simulink model "Demo_V2XStats_Intersection_1_cs"  (R2014b)
settings: Solver=FixedStepDiscrete  SolverMode=SingleTasking  StartTime=0.0  StopTime=10  FixedStep=1/20  RelTol=1e-3
PreLoadFcn:
  | mbxruntime.callbacks.PreLoadFcn(bdroot);
  | check_NUTS_defined
  | model_closed = 0;
  | assignin('base',['model_closed_' bdroot],false);
PostLoadFcn:
  | mbxruntime.callbacks.PostLoadFcn(bdroot);
InitFcn:
  | mbxruntime.callbacks.InitFcn(bdroot);
StartFcn:
  | mbxruntime.callbacks.StartFcn(bdroot);
StopFcn:
  | mbxruntime.callbacks.StopFcn(bdroot);;
  | 
  | PostProcessing
  | 
model workspace: external: MAT-File .\Demo_V2XStats_Intersection_1_cs_hws.mat (data not in the file)
undefined symbols (not defined in the file or in its folder): InitializeBus, mbxruntime, tabledata
undefined symbols (not defined in the file): Demo_V2XStats_Intersection_1_cs_022fa72960d02a99, Demo_V2XStats_Intersection_1_cs_0667b7440011464a, Demo_V2XStats_Intersection_1_cs_0a717f3b1f82dce8, Demo_V2XStats_Intersection_1_cs_1912d0ac773e0614, Demo_V2XStats_Intersection_1_cs_1b4820430dd12493, Demo_V2XStats_Intersection_1_cs_3bba87328ee67e0a, Demo_V2XStats_Intersection_1_cs_467d7b57b3557fc2, Demo_V2XStats_Intersection_1_cs_534bad308c560994, Demo_V2XStats_Intersection_1_cs_58d6839509a0e403, Demo_V2XStats_Intersection_1_cs_7e2090151d7b4087, Demo_V2XStats_Intersection_1_cs_9888c4f7e8bf41a4, Demo_V2XStats_Intersection_1_cs_a103b1f27004d7b9, Demo_V2XStats_Intersection_1_cs_dde6e9b2bb85eae6, Demo_V2XStats_Intersection_1_cs_fcdd4688b7d5d124
libraries: simulink x5, PreScanSimulinkLibrary x4, PreScanUsefulBlocks x1, simulink_extras x1
(part 2 of 3)

== system Demo_V2XStats_Intersection_1_cs/Synchronizer ==
  Bus Selector1 : BusSelector  OutputSignals=FederateStopped
  Stop Simulation : Stop
  sfun_Synchronizer : S-Function  FunctionName=sfun_Synchronizer  Parameters=SampleTime  EnableBusSupport=off  mask(Legacy Function){SFunctionSpec=void prescan_synchronizer_outputFcn(void ** work1, PRESCAN_SYNCHRONIZEDATA y1[1]), SampleTime=TimeStep, ShowSpec=on}
      mask prompts: SampleTime "Sample time (-1 for inherited):"; ShowSpec "Display function specification"
      mask help:
      | This block allows you to call the legacy functions specified by the following Legacy Code Tool definition:
      | def.SFunctionName = 'sfun_Synchronizer';
      | def.OutputFcnSpec = 'void prescan_synchronizer_outputFcn(void ** work1, PRESCAN_SYNCHRONIZEDATA y1[1])';
      | def.StartFcnSpec = 'void prescan_synchronizer_startFcn(void ** work1)';
      | def.TerminateFcnSpec = 'void prescan_synchronizer_terminateFcn(void ** work1)';
      | def.HeaderFiles = {'prescan_synchronizer_data.h'};
      | def.HostLibFiles = {'sensorinterfaced.lib'};
      | def.IncPaths = {'src', 'C:\prescandev\vislibrary\vis\..\pimp\include\sensors\InterfaceRTW'};
      | def.SrcPaths = {'src'};
      | def.LibPaths = {'C:\\prescandev\\vislibrary_build\lib'};
      | def.SampleTime = 'parameterized';
      | def.Options.language = 'C';
      mask Help: <p>This block was generated automatically by the Legacy Code Tool. For detailed help on this tool, call<a href="matlab:legacy_code('help')"> legacy_code('help')</a>.</p>
      mask Callback ShowSpec:
      | if strcmp(get_param(gcbh, 'ShowSpec'), 'on')
      |   set_param(gcbh, 'MaskDisplay', sprintf('fprintf(''%s'');', get_param(gcbh, 'SFunctionSpec')));
      | else
      |   set_param(gcbh, 'MaskDisplay', sprintf('fprintf(''%s'');', get_param(gcbh, 'FunctionName')));
      | end
      mask Display: fprintf('void prescan_synchronizer_outputFcn(void ** work1, PRESCAN_SYNCHRONIZEDATA y1[1])');
  wires:
  Bus Selector1/1 -> Stop Simulation/1  "<FederateStopped>"
  sfun_Synchronizer/1 -> Bus Selector1/1

== system Demo_V2XStats_Intersection_1_cs/V2X_Rx2816_CAM_Receiver ==
  Sensor : S-Function  LoadFcn=InitializeBus('CAM')  FunctionName=sfun_V2X_CAM_Receiver  Parameters=sensorID, parentID, maxMessages, timestep  EnableBusSupport=off  mask(V2X CAM Receiver Block){sensorID=2816, parentID=7, maxMessages=1, timestep=1/20}
      mask prompts: sensorID "Receiver ID"; parentID "Parent ID"; maxMessages "Maximum number of messages"; timestep "MATLAB timestep:"
      mask help: V2X Block receiving a CAM message
      mask Display: image(imread('V2XR_grayscale.png'))
  V2X_Rx2816_CAM_Receiver : Outport  Tag=outport/plugin/sfun_V2X_CAM_Receiver
  wires:
  Sensor/1 -> V2X_Rx2816_CAM_Receiver/1

== system Demo_V2XStats_Intersection_1_cs/V2X_Tx2817_CAM_Transmitter ==
  V2X_Tx2817_CAM_Transmitter : Inport  Tag=inport/plugin/sfun_V2X_CAM_Transmitter  BusOutputAsStruct=on
  Actuator : S-Function  FunctionName=sfun_V2X_CAM_Transmitter  Parameters=sensorID, parentID, timestep  EnableBusSupport=off  mask(V2X CAM Transmitter Block){sensorID=2817, parentID=10, timestep=1/20}
      mask prompts: sensorID "Transmitter ID"; parentID "Parent ID"; timestep "MATLAB timestep:"
      mask help: V2X Block transmitting a CAM message
      mask Display: image(imread('V2XT_grayscale.png'))
  wires:
  V2X_Tx2817_CAM_Transmitter/1 -> Actuator/1

== system Demo_V2XStats_Intersection_1_cs/VISUColorRegion_Lower_Body_Male_Regular_wSuitcase_1 ==
  VISUColorRegion_Lower_Body_Male_Regular_wSuitcase_1 : Inport  Tag=inport/ColorRegion  OutDataTypeStr=Bus: PRESCAN_COLOR_DATA  PortDimensions=1  SampleTime=1/20  BusOutputAsStruct=on
  Actuator : S-Function  FunctionName=sfun_ColorActuator  Parameters=mbxruntime.parameters.convert(UniqueID), mbxruntime.parameters.convert(WorldModelSubPath),tabledata, TimeStep  EnableBusSupport=off  mask(PreScan Sink Block: VisuTextureColor){UniqueID=2658, WorldModelSubPath=/recolorRegion:name=Lower Body/targetColor, TimeStep=1/20}
      mask prompts: UniqueID "Parent Unique Identifier (auto-generated)"; WorldModelSubPath "WM SubPath(auto-generated)"; TimeStep "Simulink time step"
      mask help:
      | The VisuTextureColor block provides a way to adapt the color of a vehicle.
      |
      | For more information, please click Help.
      mask init:
      | [tabledata] = mbxruntime.parameters.table(UniqueID,WorldModelSubPath);
      mask Help: eval('openHelp(230)')
      mask Display: image(imread('TextureColor.png'))
  wires:
  VISUColorRegion_Lower_Body_Male_Regular_wSuitcase_1/1 -> Actuator/1

== system Demo_V2XStats_Intersection_1_cs/VISUColorRegion_Shoes_Male_Regular_wSuitcase_1 ==
  VISUColorRegion_Shoes_Male_Regular_wSuitcase_1 : Inport  Tag=inport/ColorRegion  OutDataTypeStr=Bus: PRESCAN_COLOR_DATA  PortDimensions=1  SampleTime=1/20  BusOutputAsStruct=on
  Actuator : S-Function  FunctionName=sfun_ColorActuator  Parameters=mbxruntime.parameters.convert(UniqueID), mbxruntime.parameters.convert(WorldModelSubPath),tabledata, TimeStep  EnableBusSupport=off  mask(PreScan Sink Block: VisuTextureColor){UniqueID=2658, WorldModelSubPath=/recolorRegion:name=Shoes/targetColor, TimeStep=1/20}
      mask prompts: UniqueID "Parent Unique Identifier (auto-generated)"; WorldModelSubPath "WM SubPath(auto-generated)"; TimeStep "Simulink time step"
      mask help:
      | The VisuTextureColor block provides a way to adapt the color of a vehicle.
      |
      | For more information, please click Help.
      mask init:
      | [tabledata] = mbxruntime.parameters.table(UniqueID,WorldModelSubPath);
      mask Help: eval('openHelp(230)')
      mask Display: image(imread('TextureColor.png'))
  wires:
  VISUColorRegion_Shoes_Male_Regular_wSuitcase_1/1 -> Actuator/1

== system Demo_V2XStats_Intersection_1_cs/VISUColorRegion_Upper_Body_Male_Regular_wSuitcase_1 ==
  VISUColorRegion_Upper_Body_Male_Regular_wSuitcase_1 : Inport  Tag=inport/ColorRegion  OutDataTypeStr=Bus: PRESCAN_COLOR_DATA  PortDimensions=1  SampleTime=1/20  BusOutputAsStruct=on
  Actuator : S-Function  FunctionName=sfun_ColorActuator  Parameters=mbxruntime.parameters.convert(UniqueID), mbxruntime.parameters.convert(WorldModelSubPath),tabledata, TimeStep  EnableBusSupport=off  mask(PreScan Sink Block: VisuTextureColor){UniqueID=2658, WorldModelSubPath=/recolorRegion:name=Upper Body/targetColor, TimeStep=1/20}
      mask prompts: UniqueID "Parent Unique Identifier (auto-generated)"; WorldModelSubPath "WM SubPath(auto-generated)"; TimeStep "Simulink time step"
      mask help:
      | The VisuTextureColor block provides a way to adapt the color of a vehicle.
      |
      | For more information, please click Help.
      mask init:
      | [tabledata] = mbxruntime.parameters.table(UniqueID,WorldModelSubPath);
      mask Help: eval('openHelp(230)')
      mask Display: image(imread('TextureColor.png'))
  wires:
  VISUColorRegion_Upper_Body_Male_Regular_wSuitcase_1/1 -> Actuator/1

== system Demo_V2XStats_Intersection_1_cs/Male_Regular_wSuitcase_1/Animation ==
  In1 : Inport
  Bus Creator : BusCreator  Inputs=2  OutDataTypeStr=Bus: PRESCAN_ANIMACTUATORDATA  NonVirtualBus=on
  Bus Selector : BusSelector  OutputSignals=VelocityX,VelocityY,VelocityZ
  Mux : Mux  Inputs=3
  animation mode : Subsystem
  elapsed track : Subsystem
  Out1 : Outport
  wires:
  animation mode/1(mode) -> Bus Creator/1  "Index"
  Bus Creator/1 -> Out1/1
  In1/1 -> Bus Selector/1
  elapsed track/1(s) -> Bus Creator/2  "Time"
  Bus Selector/3 -> Mux/3  "<VelocityZ>"
  Bus Selector/2 -> Mux/2  "<VelocityY>"
  Bus Selector/1 -> Mux/1  "<VelocityX>"
  Mux/1 -> animation mode/1(vel), elapsed track/1(vel)

== system Demo_V2XStats_Intersection_1_cs/Male_Regular_wSuitcase_1/Dynamics_Empty ==
  note: For state mode 'Dynamic' positions
      | are not taken into account, as they
      | are computed by integrating velocity.
      | Click annotation for Help.
  note: For state mode 'Dynamic' positions
      | are not taken into account, as they
      | are computed by integrating velocity.
      | Click annotation for Help.
  Ground_{1..9} (9 alike) : Ground
  MuxState : Subsystem  Tag=mux/State  mask(Empty Dynamics State Block){positioningmode=on, TimeStep=1/20}
      mask prompts: positioningmode "Positioning Mode"; TimeStep "Auto Assigned: Time Step [s]"
      mask help:
      | Build the state of an actor based on user input.
      | The user can either use positioning mode or dynamics mode.
      | - When using positioning mode the position and orientation of the actor are set directly based on the input. Expected input is relative to the initial position and orientation of the actor. It's also possible to specify the velocity of the actor, though this input isn't used, only passed on.
      | - When using dynamics mode the position input is ignored. Expected input is velocity and orientation. The velocity is relative the current orientation of the actor, while orientation is relative to its initial orientation. The position of the actor is calculated based on the velocity and orientation given.
      settings: DeleteFcn=PreScanBlockDeleteFcn;
  STATE_Male_Regular_wSuitcase_1 : Subsystem  Tag=mux/StatePort  Priority=0  LoadFcn=load PrescanStateActuatorData  mask(PreScan Sink Block: State){x0=Demo_V2XStats_Intersection_1_cs_9888c4f7e8bf41a4, y0=Demo_V2XStats_Intersection_1_cs_0667b7440011464a, z0=Demo_V2XStats_Intersection_1_cs_1b4820430dd12493, Roll0=Demo_V2XStats_Intersection_1_cs_dde6e9b2bb85eae6, Pitch0=Demo_V2XStats_Intersection_1_cs_1912d0ac773e0614, Yaw0=Demo_V2XStats_Intersection_1_cs_58d6839509a0e403, TimeStep=1/20}
      mask prompts: x0 "Ini x-position VEHICLE wrt GLOBAL axis system [m]"; y0 "Ini y-position VEHICLE wrt GLOBAL axis system [m]"; z0 "Ini z-position VEHICLE wrt GLOBAL axis system [m]"; Roll0 "Ini roll-angle BODY wrt VEHICLE axis system [deg]"; Pitch0 "Ini pitch-angle BODY wrt VEHICLE axis system [deg]"; Yaw0 "Ini yaw-angle VEHICLE wrt GLOBAL axis system [deg]"; TimeStep "Auto-Assigned: Upload Period [s]"
      mask help:
      | The Actor State contains a vector signal of size (9x1), containing the following signals:
      |
      | -  Position                  (x,y,z)                                     [m]
      | -  Velocity                  (vx,vy,vz)                               [m/s]
      | -  Angles                    (Roll, Pitch, Yaw)                   [rad]
      |
      | The Actor state is defined in the global axis system.
      | The state is superponed on the Initial position defined in the GUI.
      |
      | For more information, please click Help.
      settings: DeleteFcn=PreScanBlockDeleteFcn;
      mask Help: eval('openHelp(222)')
      mask Display: image(imread('State.png'))
  State : Outport  Tag=outport/StateOutport  SampleTime=1/20
  wires:
  STATE_Male_Regular_wSuitcase_1/1(StateBus) -> State/1
  MuxState/1(state) -> STATE_Male_Regular_wSuitcase_1/1(State)
  Ground_1/1 -> MuxState/1(x [m])
  Ground_2/1 -> MuxState/2(y [m])
  Ground_3/1 -> MuxState/3(z [m])
  Ground_4/1 -> MuxState/4(dx [m/s])
  Ground_5/1 -> MuxState/5(dy [m/s])
  Ground_6/1 -> MuxState/6(dz [m/s])
  Ground_7/1 -> MuxState/7(R [rad])
  Ground_8/1 -> MuxState/8(P [rad])
  Ground_9/1 -> MuxState/9(Y [rad])

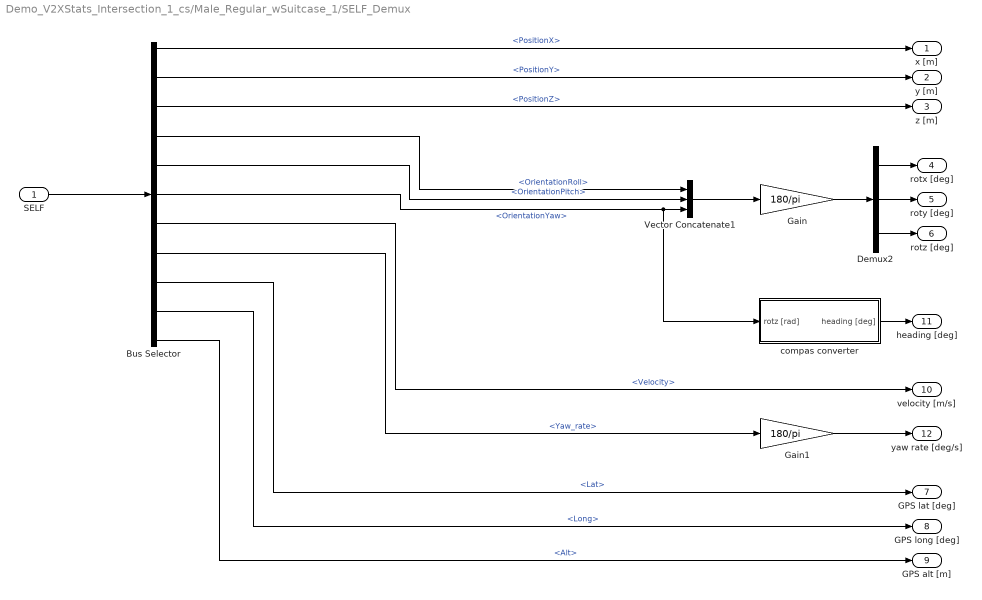
== system Demo_V2XStats_Intersection_1_cs/Male_Regular_wSuitcase_1/SELF_Demux ==
  SELF : Inport  OutDataTypeStr=Bus: PRESCAN_SELFSENSORDATA
  Bus Selector : BusSelector  OutputSignals=PositionX,PositionY,PositionZ,OrientationRoll,OrientationPitch,OrientationYaw,Velocity,Yaw_rate,Lat,Long,Alt
  Demux2 : Demux  Outputs=3
  Gain : Gain  Gain=180/pi
  Gain1 : Gain  Gain=180/pi
  Vector Concatenate1 : Concatenate  NumInputs=3
  compas converter : Subsystem
  x [m] : Outport
  y [m] : Outport  Port=2
  z [m] : Outport  Port=3
  rotx [deg] : Outport  Port=4
  roty [deg] : Outport  Port=5
  rotz [deg] : Outport  Port=6
  GPS lat [deg] : Outport  Port=7
  GPS long [deg] : Outport  Port=8
  GPS alt [m] : Outport  Port=9
  velocity [m/s] : Outport  Port=10
  heading [deg] : Outport  Port=11
  yaw rate [deg/s] : Outport  Port=12
  wires:
  Bus Selector/11 -> GPS alt [m]/1  "<Alt>"
  Bus Selector/10 -> GPS long [deg]/1  "<Long>"
  Bus Selector/9 -> GPS lat [deg]/1  "<Lat>"
  Bus Selector/8 -> Gain1/1  "<Yaw_rate>"
  Bus Selector/7 -> velocity [m/s]/1  "<Velocity>"
  Bus Selector/6 -> compas converter/1(rotz [rad]), Vector Concatenate1/3  "<OrientationYaw>"
  Bus Selector/5 -> Vector Concatenate1/2  "<OrientationPitch>"
  Bus Selector/4 -> Vector Concatenate1/1  "<OrientationRoll>"
  Vector Concatenate1/1 -> Gain/1
  Bus Selector/3 -> z [m]/1  "<PositionZ>"
  Bus Selector/2 -> y [m]/1  "<PositionY>"
  Bus Selector/1 -> x [m]/1  "<PositionX>"
  SELF/1 -> Bus Selector/1
  Gain/1 -> Demux2/1
  Demux2/1 -> rotx [deg]/1
  Demux2/2 -> roty [deg]/1
  Demux2/3 -> rotz [deg]/1
  compas converter/1(heading [deg]) -> heading [deg]/1
  Gain1/1 -> yaw rate [deg/s]/1

== system Demo_V2XStats_Intersection_1_cs/Male_Regular_wSuitcase_1/VISUColorRegion_Lower_Body_Mux ==
  RGB [-,-,-] : Inport
  Bus Creator : BusCreator  OutDataTypeStr=Bus: PRESCAN_COLOR_DATA  NonVirtualBus=on
  Constant : Constant  Value=255  OutDataTypeStr=uint8
  Data Type Conversion : DataTypeConversion  OutDataTypeStr=uint8
  Data Type Conversion1 : DataTypeConversion  OutDataTypeStr=uint8
  Data Type Conversion2 : DataTypeConversion  OutDataTypeStr=uint8
  Demux : Demux  Outputs=3
  ColorRegion : Outport  OutDataTypeStr=Bus: PRESCAN_COLOR_DATA  PortDimensions=1
  wires:
  Constant/1 -> Bus Creator/4  "A"
  Data Type Conversion2/1 -> Bus Creator/3  "B"
  Data Type Conversion1/1 -> Bus Creator/2  "G"
  Data Type Conversion/1 -> Bus Creator/1  "R"
  Demux/3 -> Data Type Conversion2/1  "B"
  Demux/2 -> Data Type Conversion1/1  "G"
  Demux/1 -> Data Type Conversion/1  "R"
  RGB [-,-,-]/1 -> Demux/1
  Bus Creator/1 -> ColorRegion/1

== system Demo_V2XStats_Intersection_1_cs/Male_Regular_wSuitcase_1/VISUColorRegion_Shoes_Mux ==
  RGB [-,-,-] : Inport
  Bus Creator : BusCreator  OutDataTypeStr=Bus: PRESCAN_COLOR_DATA  NonVirtualBus=on
  Constant : Constant  Value=255  OutDataTypeStr=uint8
  Data Type Conversion : DataTypeConversion  OutDataTypeStr=uint8
  Data Type Conversion1 : DataTypeConversion  OutDataTypeStr=uint8
  Data Type Conversion2 : DataTypeConversion  OutDataTypeStr=uint8
  Demux : Demux  Outputs=3
  ColorRegion : Outport  OutDataTypeStr=Bus: PRESCAN_COLOR_DATA  PortDimensions=1
  wires:
  Constant/1 -> Bus Creator/4  "A"
  Data Type Conversion2/1 -> Bus Creator/3  "B"
  Data Type Conversion1/1 -> Bus Creator/2  "G"
  Data Type Conversion/1 -> Bus Creator/1  "R"
  Demux/3 -> Data Type Conversion2/1  "B"
  Demux/2 -> Data Type Conversion1/1  "G"
  Demux/1 -> Data Type Conversion/1  "R"
  RGB [-,-,-]/1 -> Demux/1
  Bus Creator/1 -> ColorRegion/1

== system Demo_V2XStats_Intersection_1_cs/Male_Regular_wSuitcase_1/VISUColorRegion_Upper_Body_Mux ==
  RGB [-,-,-] : Inport
  Bus Creator : BusCreator  OutDataTypeStr=Bus: PRESCAN_COLOR_DATA  NonVirtualBus=on
  Constant : Constant  Value=255  OutDataTypeStr=uint8
  Data Type Conversion : DataTypeConversion  OutDataTypeStr=uint8
  Data Type Conversion1 : DataTypeConversion  OutDataTypeStr=uint8
  Data Type Conversion2 : DataTypeConversion  OutDataTypeStr=uint8
  Demux : Demux  Outputs=3
  ColorRegion : Outport  OutDataTypeStr=Bus: PRESCAN_COLOR_DATA  PortDimensions=1
  wires:
  Constant/1 -> Bus Creator/4  "A"
  Data Type Conversion2/1 -> Bus Creator/3  "B"
  Data Type Conversion1/1 -> Bus Creator/2  "G"
  Data Type Conversion/1 -> Bus Creator/1  "R"
  Demux/3 -> Data Type Conversion2/1  "B"
  Demux/2 -> Data Type Conversion1/1  "G"
  Demux/1 -> Data Type Conversion/1  "R"
  RGB [-,-,-]/1 -> Demux/1
  Bus Creator/1 -> ColorRegion/1

== system Demo_V2XStats_Intersection_1_cs/Mazda_RX8_1/Dynamics_Empty ==
  note: For state mode 'Dynamic' positions
      | are not taken into account, as they
      | are computed by integrating velocity.
      | Click annotation for Help.
  note: For state mode 'Dynamic' positions
      | are not taken into account, as they
      | are computed by integrating velocity.
      | Click annotation for Help.
  Ground_{1..9} (9 alike) : Ground
  MuxState : Subsystem  Tag=mux/State  mask(Empty Dynamics State Block){positioningmode=on, TimeStep=1/20}
      mask prompts: positioningmode "Positioning Mode"; TimeStep "Auto Assigned: Time Step [s]"
      mask help:
      | Build the state of an actor based on user input.
      | The user can either use positioning mode or dynamics mode.
      | - When using positioning mode the position and orientation of the actor are set directly based on the input. Expected input is relative to the initial position and orientation of the actor. It's also possible to specify the velocity of the actor, though this input isn't used, only passed on.
      | - When using dynamics mode the position input is ignored. Expected input is velocity and orientation. The velocity is relative the current orientation of the actor, while orientation is relative to its initial orientation. The position of the actor is calculated based on the velocity and orientation given.
      settings: DeleteFcn=PreScanBlockDeleteFcn;
  STATE_Mazda_RX8_1 : Subsystem  Tag=mux/StatePort  Priority=0  LoadFcn=load PrescanStateActuatorData  mask(PreScan Sink Block: State){x0=Demo_V2XStats_Intersection_1_cs_7e2090151d7b4087, y0=Demo_V2XStats_Intersection_1_cs_534bad308c560994, z0=Demo_V2XStats_Intersection_1_cs_467d7b57b3557fc2, Roll0=Demo_V2XStats_Intersection_1_cs_0a717f3b1f82dce8, Pitch0=Demo_V2XStats_Intersection_1_cs_3bba87328ee67e0a, Yaw0=Demo_V2XStats_Intersection_1_cs_022fa72960d02a99, TimeStep=1/20}
      mask prompts: x0 "Ini x-position VEHICLE wrt GLOBAL axis system [m]"; y0 "Ini y-position VEHICLE wrt GLOBAL axis system [m]"; z0 "Ini z-position VEHICLE wrt GLOBAL axis system [m]"; Roll0 "Ini roll-angle BODY wrt VEHICLE axis system [deg]"; Pitch0 "Ini pitch-angle BODY wrt VEHICLE axis system [deg]"; Yaw0 "Ini yaw-angle VEHICLE wrt GLOBAL axis system [deg]"; TimeStep "Auto-Assigned: Upload Period [s]"
      mask help:
      | The Actor State contains a vector signal of size (9x1), containing the following signals:
      |
      | -  Position                  (x,y,z)                                     [m]
      | -  Velocity                  (vx,vy,vz)                               [m/s]
      | -  Angles                    (Roll, Pitch, Yaw)                   [rad]
      |
      | The Actor state is defined in the global axis system.
      | The state is superponed on the Initial position defined in the GUI.
      |
      | For more information, please click Help.
      settings: DeleteFcn=PreScanBlockDeleteFcn;
      mask Help: eval('openHelp(222)')
      mask Display: image(imread('State.png'))
  State : Outport  Tag=outport/StateOutport  SampleTime=1/20
  wires:
  STATE_Mazda_RX8_1/1(StateBus) -> State/1
  MuxState/1(state) -> STATE_Mazda_RX8_1/1(State)
  Ground_1/1 -> MuxState/1(x [m])
  Ground_2/1 -> MuxState/2(y [m])
  Ground_3/1 -> MuxState/3(z [m])
  Ground_4/1 -> MuxState/4(dx [m/s])
  Ground_5/1 -> MuxState/5(dy [m/s])
  Ground_6/1 -> MuxState/6(dz [m/s])
  Ground_7/1 -> MuxState/7(R [rad])
  Ground_8/1 -> MuxState/8(P [rad])
  Ground_9/1 -> MuxState/9(Y [rad])

== system Demo_V2XStats_Intersection_1_cs/Mazda_RX8_1/Retreive car data using ID info ==
  note: id=4
  note: id=4
  note: Assumption:
      | All vehicles are visible all time.
      | So the data can be ordered by using the id order.
      | id=0 (meaning no detection) does not exist
  Lat_detected : Inport
  Lon_detected : Inport  Port=2
  Alt_detected : Inport  Port=3
  Intention_detected : Inport  Port=4
  Heading_detected : Inport  Port=5
  Complex to Magnitude-Angle1 : ComplexToMagnitudeAngle
  Demux1 : Demux  Outputs=2
  GPS2xyz : PreScanUsefulBlocks/GPS2xyz  CoordinateCount=1  GPS_base=[0 0 0]
  Mux : Mux
  Mux3 : Mux  Inputs=3
  Radians to Degrees : simulink_extras/Transformations/Radians to Degrees
  Real-Imag to Complex1 : RealImagToComplex
  Selector : Selector  Indices=[1 2]
  Cabstar : Outport
  wires:
  Heading_detected/1 -> Mux/4  "heading"
  Intention_detected/1 -> Mux/3  "intention"
  Alt_detected/1 -> Mux3/3
  Lon_detected/1 -> Mux3/2
  Lat_detected/1 -> Mux3/1
  Mux/1 -> Cabstar/1
  Mux3/1 -> GPS2xyz/1
  Demux1/2 -> Real-Imag to Complex1/2
  Demux1/1 -> Real-Imag to Complex1/1
  Real-Imag to Complex1/1 -> Complex to Magnitude-Angle1/1
  Complex to Magnitude-Angle1/2 -> Radians to Degrees/1
  Radians to Degrees/1 -> Mux/2  "angle"
  Complex to Magnitude-Angle1/1 -> Mux/1  "range"
  Selector/1 -> Demux1/1
  GPS2xyz/1 -> Selector/1

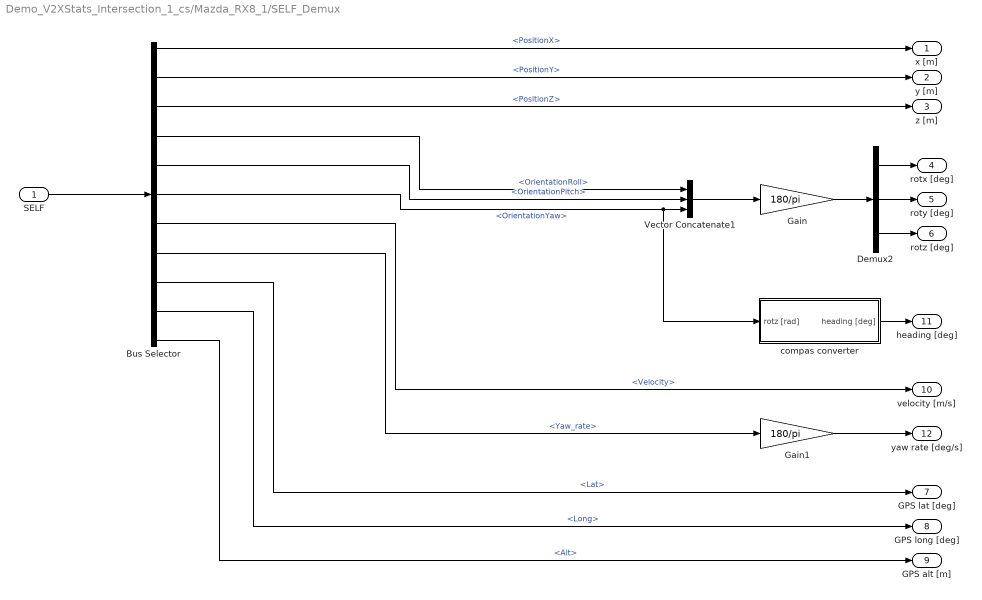
== system Demo_V2XStats_Intersection_1_cs/Mazda_RX8_1/SELF_Demux ==
  SELF : Inport  OutDataTypeStr=Bus: PRESCAN_SELFSENSORDATA
  Bus Selector : BusSelector  OutputSignals=PositionX,PositionY,PositionZ,OrientationRoll,OrientationPitch,OrientationYaw,Velocity,Yaw_rate,Lat,Long,Alt
  Demux2 : Demux  Outputs=3
  Gain : Gain  Gain=180/pi
  Gain1 : Gain  Gain=180/pi
  Vector Concatenate1 : Concatenate  NumInputs=3
  compas converter : Subsystem
  x [m] : Outport
  y [m] : Outport  Port=2
  z [m] : Outport  Port=3
  rotx [deg] : Outport  Port=4
  roty [deg] : Outport  Port=5
  rotz [deg] : Outport  Port=6
  GPS lat [deg] : Outport  Port=7
  GPS long [deg] : Outport  Port=8
  GPS alt [m] : Outport  Port=9
  velocity [m/s] : Outport  Port=10
  heading [deg] : Outport  Port=11
  yaw rate [deg/s] : Outport  Port=12
  wires:
  Bus Selector/11 -> GPS alt [m]/1  "<Alt>"
  Bus Selector/10 -> GPS long [deg]/1  "<Long>"
  Bus Selector/9 -> GPS lat [deg]/1  "<Lat>"
  Bus Selector/8 -> Gain1/1  "<Yaw_rate>"
  Bus Selector/7 -> velocity [m/s]/1  "<Velocity>"
  Bus Selector/6 -> compas converter/1(rotz [rad]), Vector Concatenate1/3  "<OrientationYaw>"
  Bus Selector/5 -> Vector Concatenate1/2  "<OrientationPitch>"
  Bus Selector/4 -> Vector Concatenate1/1  "<OrientationRoll>"
  Vector Concatenate1/1 -> Gain/1
  Bus Selector/3 -> z [m]/1  "<PositionZ>"
  Bus Selector/2 -> y [m]/1  "<PositionY>"
  Bus Selector/1 -> x [m]/1  "<PositionX>"
  SELF/1 -> Bus Selector/1
  Gain/1 -> Demux2/1
  Demux2/1 -> rotx [deg]/1
  Demux2/2 -> roty [deg]/1
  Demux2/3 -> rotz [deg]/1
  compas converter/1(heading [deg]) -> heading [deg]/1
  Gain1/1 -> yaw rate [deg/s]/1

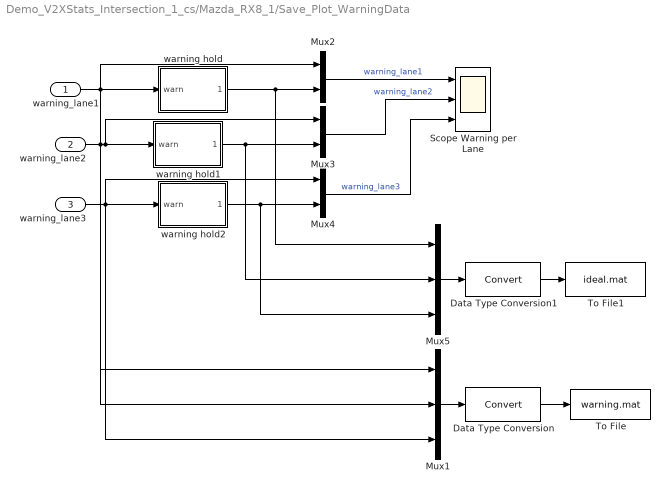
== system Demo_V2XStats_Intersection_1_cs/Mazda_RX8_1/Save_Plot_WarningData ==
  warning_lane1 : Inport
  warning_lane2 : Inport  Port=2
  warning_lane3 : Inport  Port=3
  Data Type Conversion : DataTypeConversion
  Data Type Conversion1 : DataTypeConversion
  Mux1 : Mux  Inputs=3
  Mux2 : Mux  Inputs=2
  Mux3 : Mux  Inputs=2
  Mux4 : Mux  Inputs=2
  Mux5 : Mux  Inputs=3
  Scope Warning per Lane : Scope  NumInputPorts=3
      settings: YMin=-5~-5~-5  YMax=5~5~5
  To File : ToFile  Filename=warning.mat  MatrixName=warning
  To File1 : ToFile  Filename=ideal.mat  MatrixName=ideal
  warning hold : Subsystem
  warning hold1 : Subsystem
  warning hold2 : Subsystem
  wires:
  Mux1/1 -> Data Type Conversion/1
  warning_lane3/1 -> Mux1/3, warning hold2/1(warn), Mux4/1
  warning_lane2/1 -> Mux1/2, warning hold1/1(warn), Mux3/1
  warning_lane1/1 -> Mux1/1, Mux2/1, warning hold/1(warn)
  Data Type Conversion1/1 -> To File1/1
  Mux5/1 -> Data Type Conversion1/1
  Data Type Conversion/1 -> To File/1
  Mux4/1 -> Scope Warning per Lane/3  "warning_lane3"
  Mux3/1 -> Scope Warning per Lane/2  "warning_lane2"
  Mux2/1 -> Scope Warning per Lane/1  "warning_lane1"
  warning hold2/1(warning) -> Mux5/3, Mux4/2
  warning hold1/1(warning) -> Mux5/2, Mux3/2
  warning hold/1(warning) -> Mux5/1, Mux2/2

== system Demo_V2XStats_Intersection_1_cs/Mazda_RX8_1/V2x_TC_GUI1 ==
  warning : Inport
  message : Inport  Port=2
  velocity : Inport  Port=3
  Constant : Constant  Value=800
  Constant2 : Constant  Value=0
  Constant3 : Constant  Value=0
  Data Type Conversion : DataTypeConversion
  Data Type Conversion1 : DataTypeConversion
  Detect Change : simulink/Logic and Bit Operations/Detect Change  vinit=0  InputProcessing=Inherited  OutDataTypeStr=uint8
  V2x_TC_GUI : M-S-Function  FunctionName=msfcn_V2x_TC_GUI
      mask Display:
      | port_label('input', 1, 'RPM');
      | port_label('input', 2, 'Velocity');
      | port_label('input', 3, 'Brake');
      | port_label('input', 4, 'Throttle');
      | port_label('input', 5, 'Message');
      | port_label('input', 6, 'Change');
      | port_label('input', 7, 'Warning');
  "[ms to kmh]" : Gain  Gain=3.6
  wires:
  "[ms to kmh]"/1 -> V2x_TC_GUI/2
  Constant3/1 -> V2x_TC_GUI/4
  Constant2/1 -> V2x_TC_GUI/3
  velocity/1 -> "[ms to kmh]"/1
  Constant/1 -> V2x_TC_GUI/1
  Data Type Conversion1/1 -> V2x_TC_GUI/7
  warning/1 -> Data Type Conversion1/1, Detect Change/1
  Data Type Conversion/1 -> V2x_TC_GUI/6
  Detect Change/1 -> Data Type Conversion/1
  message/1 -> V2x_TC_GUI/5

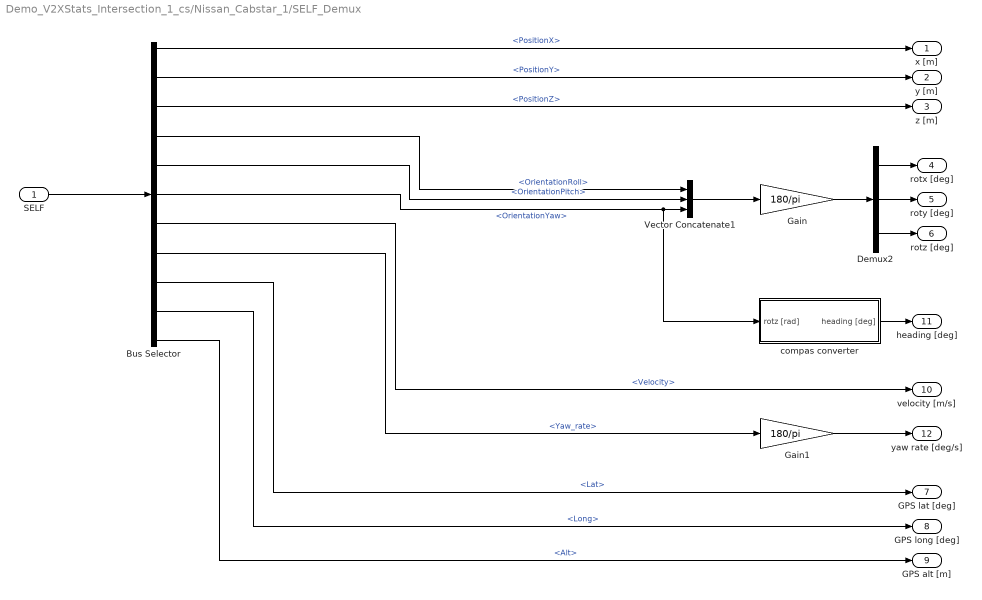
== system Demo_V2XStats_Intersection_1_cs/Nissan_Cabstar_1/SELF_Demux ==
  SELF : Inport  OutDataTypeStr=Bus: PRESCAN_SELFSENSORDATA
  Bus Selector : BusSelector  OutputSignals=PositionX,PositionY,PositionZ,OrientationRoll,OrientationPitch,OrientationYaw,Velocity,Yaw_rate,Lat,Long,Alt
  Demux2 : Demux  Outputs=3
  Gain : Gain  Gain=180/pi
  Gain1 : Gain  Gain=180/pi
  Vector Concatenate1 : Concatenate  NumInputs=3
  compas converter : Subsystem
  x [m] : Outport
  y [m] : Outport  Port=2
  z [m] : Outport  Port=3
  rotx [deg] : Outport  Port=4
  roty [deg] : Outport  Port=5
  rotz [deg] : Outport  Port=6
  GPS lat [deg] : Outport  Port=7
  GPS long [deg] : Outport  Port=8
  GPS alt [m] : Outport  Port=9
  velocity [m/s] : Outport  Port=10
  heading [deg] : Outport  Port=11
  yaw rate [deg/s] : Outport  Port=12
  wires:
  Bus Selector/11 -> GPS alt [m]/1  "<Alt>"
  Bus Selector/10 -> GPS long [deg]/1  "<Long>"
  Bus Selector/9 -> GPS lat [deg]/1  "<Lat>"
  Bus Selector/8 -> Gain1/1  "<Yaw_rate>"
  Bus Selector/7 -> velocity [m/s]/1  "<Velocity>"
  Bus Selector/6 -> compas converter/1(rotz [rad]), Vector Concatenate1/3  "<OrientationYaw>"
  Bus Selector/5 -> Vector Concatenate1/2  "<OrientationPitch>"
  Bus Selector/4 -> Vector Concatenate1/1  "<OrientationRoll>"
  Vector Concatenate1/1 -> Gain/1
  Bus Selector/3 -> z [m]/1  "<PositionZ>"
  Bus Selector/2 -> y [m]/1  "<PositionY>"
  Bus Selector/1 -> x [m]/1  "<PositionX>"
  SELF/1 -> Bus Selector/1
  Gain/1 -> Demux2/1
  Demux2/1 -> rotx [deg]/1
  Demux2/2 -> roty [deg]/1
  Demux2/3 -> rotz [deg]/1
  compas converter/1(heading [deg]) -> heading [deg]/1
  Gain1/1 -> yaw rate [deg/s]/1

== system Demo_V2XStats_Intersection_1_cs/Male_Regular_wSuitcase_1/Animation/animation mode ==
  vel : Inport
  Data Type Conversion : DataTypeConversion  OutDataTypeStr=int32
  Fcn : Fcn  Expr=u(1)^2+u(2)^2+u(3)^2
  Walking : simulink/Logic and Bit Operations/Compare To Zero  relop=~=  OutDataTypeStr=uint8  ZeroCross=off
  mode : Outport
  wires:
  Data Type Conversion/1 -> mode/1
  Walking/1 -> Data Type Conversion/1
  Fcn/1 -> Walking/1
  vel/1 -> Fcn/1

== system Demo_V2XStats_Intersection_1_cs/Male_Regular_wSuitcase_1/Animation/elapsed track ==
  vel : Inport
  Discrete-Time Integrator : DiscreteIntegrator  SampleTime=-1
  Fcn : Fcn  Expr=sqrt(u(1)^2 + u(2)^2 + u(3)^2)
  s : Outport
  wires:
  Discrete-Time Integrator/1 -> s/1
  vel/1 -> Fcn/1
  Fcn/1 -> Discrete-Time Integrator/1

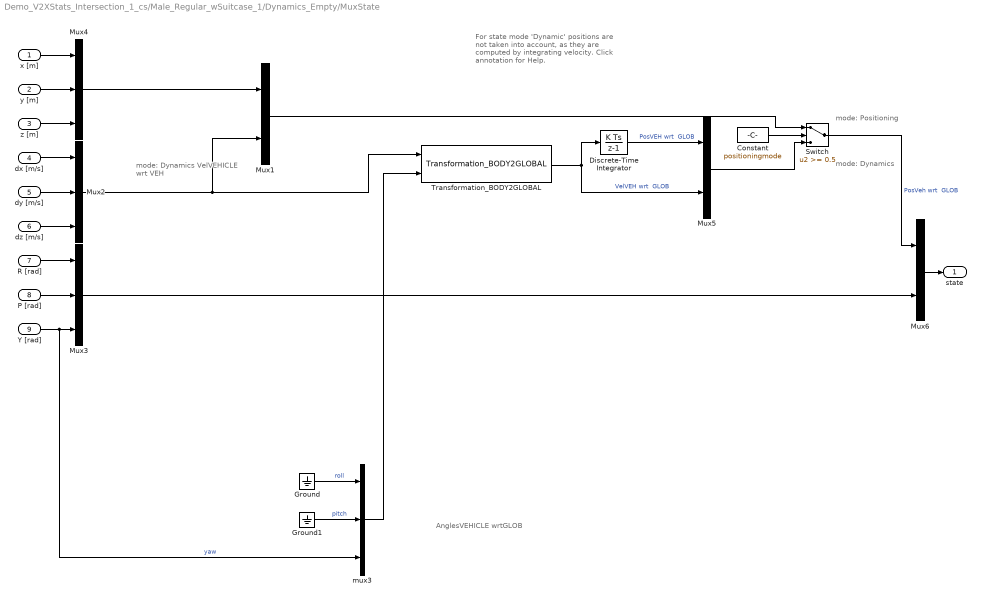
== system Demo_V2XStats_Intersection_1_cs/Male_Regular_wSuitcase_1/Dynamics_Empty/MuxState ==
  note: mode: Dynamics
  note: mode: Positioning
  note: mode: Dynamics
      | VelVEHICLE
      | wrt VEH
  note: AnglesVEHICLE
      | wrtGLOB
  note: For state mode 'Dynamic' positions
      | are not taken into account, as they
      | are computed by integrating velocity.
      | Click annotation for Help.
  x [m] : Inport  SampleTime=TimeStep
  y [m] : Inport  Port=2  SampleTime=TimeStep
  z [m] : Inport  Port=3  SampleTime=TimeStep
  dx [m/s] : Inport  Port=4  SampleTime=TimeStep
  dy [m/s] : Inport  Port=5  SampleTime=TimeStep
  dz [m/s] : Inport  Port=6  SampleTime=TimeStep
  R [rad] : Inport  Port=7  SampleTime=TimeStep
  P [rad] : Inport  Port=8  SampleTime=TimeStep
  Y [rad] : Inport  Port=9  SampleTime=TimeStep
  Constant : Constant  DisableCoverage=on  Value=positioningmode
  Discrete-Time Integrator : DiscreteIntegrator  SampleTime=TimeStep
  Ground : Ground
  Ground1 : Ground
  Mux1 : Mux  Inputs=[3 3]
  Mux2 : Mux  Inputs=3
  Mux3 : Mux  Inputs=3
  Mux4 : Mux  Inputs=3
  Mux5 : Mux  Inputs=[3 3]
  Mux6 : Mux  Inputs=[6 3]
  Switch : Switch  Threshold=0.5
  Transformation_BODY2GLOBAL : PreScanSimulinkLibrary/Simple_Vehicle_Dynamics/Chassis/MuxDynState/Transformation_BODY2GLOBAL
  mux3 : Mux  Inputs=3
  state : Outport
  wires:
  Constant/1 -> Switch/2
  Mux6/1 -> state/1
  Mux4/1 -> Mux1/1
  Mux5/1 -> Switch/3
  Mux1/1 -> Switch/1
  Switch/1 -> Mux6/1  "PosVeh wrt  GLOB"
  P [rad]/1 -> Mux3/2
  R [rad]/1 -> Mux3/1
  dz [m/s]/1 -> Mux2/3
  dy [m/s]/1 -> Mux2/2
  dx [m/s]/1 -> Mux2/1
  z [m]/1 -> Mux4/3
  y [m]/1 -> Mux4/2
  x [m]/1 -> Mux4/1
  Ground1/1 -> mux3/2  "pitch"
  Y [rad]/1 -> mux3/3, Mux3/3  "yaw"
  Mux3/1 -> Mux6/2
  Transformation_BODY2GLOBAL/1 -> Discrete-Time Integrator/1, Mux5/2  "VelVEH wrt  GLOB"
  mux3/1 -> Transformation_BODY2GLOBAL/2
  Ground/1 -> mux3/1  "roll"
  Mux2/1 -> Mux1/2, Transformation_BODY2GLOBAL/1
  Discrete-Time Integrator/1 -> Mux5/1  "PosVEH wrt  GLOB"

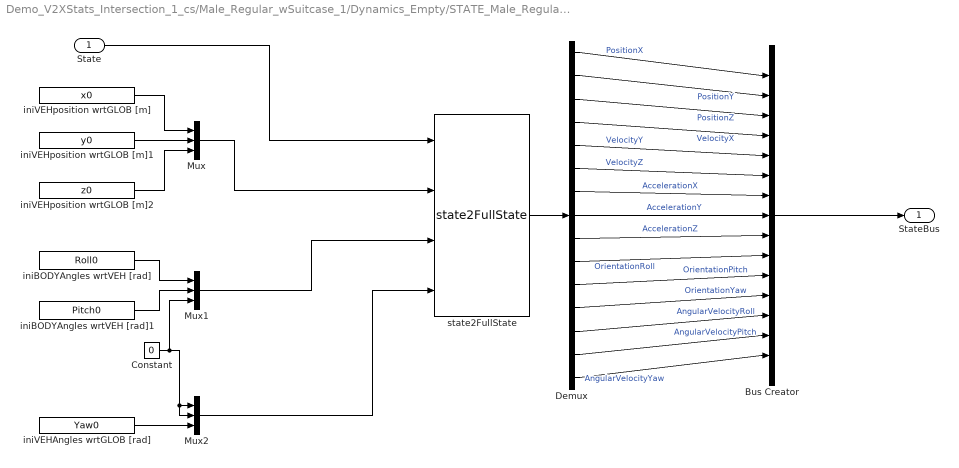
== system Demo_V2XStats_Intersection_1_cs/Male_Regular_wSuitcase_1/Dynamics_Empty/STATE_Male_Regular_wSuitcase_1 ==
  State : Inport  SampleTime=TimeStep
  Bus Creator : BusCreator  Inputs=15  OutDataTypeStr=Bus: PRESCAN_STATEACTUATORDATA  NonVirtualBus=on
  Constant : Constant  Value=0
  Demux : Demux  Outputs=15
  Mux : Mux  Inputs=3
  Mux1 : Mux  Inputs=3
  Mux2 : Mux  Inputs=3
  iniBODYAngles wrtVEH [rad] : Constant  Value=Roll0  SampleTime=TimeStep
  iniBODYAngles wrtVEH [rad]1 : Constant  Value=Pitch0  SampleTime=TimeStep
  iniVEHAngles wrtGLOB [rad] : Constant  Value=Yaw0  SampleTime=TimeStep
  iniVEHposition wrtGLOB [m] : Constant  Value=x0  SampleTime=TimeStep
  iniVEHposition wrtGLOB [m]1 : Constant  Value=y0  SampleTime=TimeStep
  iniVEHposition wrtGLOB [m]2 : Constant  Value=z0  SampleTime=TimeStep
  state2FullState : PreScanSimulinkLibrary/state2FullState  SystemSampleTime=-1
  StateBus : Outport  OutDataTypeStr=Bus: PRESCAN_STATEACTUATORDATA
  wires:
  Mux2/1 -> state2FullState/4
  iniVEHAngles wrtGLOB [rad]/1 -> Mux2/3
  Mux1/1 -> state2FullState/3
  Constant/1 -> Mux2/1, Mux2/2, Mux1/3
  iniBODYAngles wrtVEH [rad]1/1 -> Mux1/2
  iniBODYAngles wrtVEH [rad]/1 -> Mux1/1
  Mux/1 -> state2FullState/2
  iniVEHposition wrtGLOB [m]2/1 -> Mux/3
  iniVEHposition wrtGLOB [m]/1 -> Mux/1
  iniVEHposition wrtGLOB [m]1/1 -> Mux/2
  Demux/15 -> Bus Creator/15  "AngularVelocityYaw"
  Demux/14 -> Bus Creator/14  "AngularVelocityPitch"
  Demux/13 -> Bus Creator/13  "AngularVelocityRoll"
  Demux/12 -> Bus Creator/12  "OrientationYaw"
  Demux/11 -> Bus Creator/11  "OrientationPitch"
  Demux/10 -> Bus Creator/10  "OrientationRoll"
  Demux/9 -> Bus Creator/9  "AccelerationZ"
  Demux/8 -> Bus Creator/8  "AccelerationY"
  Demux/7 -> Bus Creator/7  "AccelerationX"
  Demux/6 -> Bus Creator/6  "VelocityZ"
  Demux/5 -> Bus Creator/5  "VelocityY"
  Demux/4 -> Bus Creator/4  "VelocityX"
  Demux/3 -> Bus Creator/3  "PositionZ"
  Demux/2 -> Bus Creator/2  "PositionY"
  Demux/1 -> Bus Creator/1  "PositionX"
  state2FullState/1 -> Demux/1
  State/1 -> state2FullState/1
  Bus Creator/1 -> StateBus/1

== system Demo_V2XStats_Intersection_1_cs/Male_Regular_wSuitcase_1/SELF_Demux/compas converter ==
  rotz [rad] : Inport
  cart2compas : Subsystem
  rad2deg : Gain  Gain=180/pi
  heading [deg] : Outport
  wires:
  rad2deg/1 -> cart2compas/1(Angle [deg])
  rotz [rad]/1 -> rad2deg/1
  cart2compas/1(heading [deg]) -> heading [deg]/1

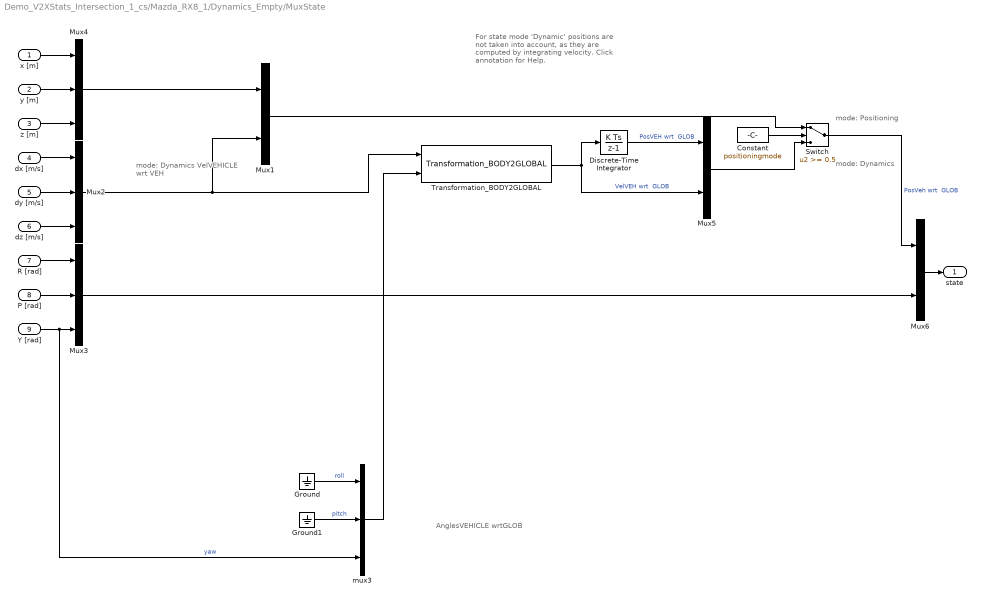
== system Demo_V2XStats_Intersection_1_cs/Mazda_RX8_1/Dynamics_Empty/MuxState ==
  note: mode: Dynamics
  note: mode: Positioning
  note: mode: Dynamics
      | VelVEHICLE
      | wrt VEH
  note: AnglesVEHICLE
      | wrtGLOB
  note: For state mode 'Dynamic' positions
      | are not taken into account, as they
      | are computed by integrating velocity.
      | Click annotation for Help.
  x [m] : Inport  SampleTime=TimeStep
  y [m] : Inport  Port=2  SampleTime=TimeStep
  z [m] : Inport  Port=3  SampleTime=TimeStep
  dx [m/s] : Inport  Port=4  SampleTime=TimeStep
  dy [m/s] : Inport  Port=5  SampleTime=TimeStep
  dz [m/s] : Inport  Port=6  SampleTime=TimeStep
  R [rad] : Inport  Port=7  SampleTime=TimeStep
  P [rad] : Inport  Port=8  SampleTime=TimeStep
  Y [rad] : Inport  Port=9  SampleTime=TimeStep
  Constant : Constant  DisableCoverage=on  Value=positioningmode
  Discrete-Time Integrator : DiscreteIntegrator  SampleTime=TimeStep
  Ground : Ground
  Ground1 : Ground
  Mux1 : Mux  Inputs=[3 3]
  Mux2 : Mux  Inputs=3
  Mux3 : Mux  Inputs=3
  Mux4 : Mux  Inputs=3
  Mux5 : Mux  Inputs=[3 3]
  Mux6 : Mux  Inputs=[6 3]
  Switch : Switch  Threshold=0.5
  Transformation_BODY2GLOBAL : PreScanSimulinkLibrary/Simple_Vehicle_Dynamics/Chassis/MuxDynState/Transformation_BODY2GLOBAL
  mux3 : Mux  Inputs=3
  state : Outport
  wires:
  Constant/1 -> Switch/2
  Mux6/1 -> state/1
  Mux4/1 -> Mux1/1
  Mux5/1 -> Switch/3
  Mux1/1 -> Switch/1
  Switch/1 -> Mux6/1  "PosVeh wrt  GLOB"
  P [rad]/1 -> Mux3/2
  R [rad]/1 -> Mux3/1
  dz [m/s]/1 -> Mux2/3
  dy [m/s]/1 -> Mux2/2
  dx [m/s]/1 -> Mux2/1
  z [m]/1 -> Mux4/3
  y [m]/1 -> Mux4/2
  x [m]/1 -> Mux4/1
  Ground1/1 -> mux3/2  "pitch"
  Y [rad]/1 -> mux3/3, Mux3/3  "yaw"
  Mux3/1 -> Mux6/2
  Transformation_BODY2GLOBAL/1 -> Discrete-Time Integrator/1, Mux5/2  "VelVEH wrt  GLOB"
  mux3/1 -> Transformation_BODY2GLOBAL/2
  Ground/1 -> mux3/1  "roll"
  Mux2/1 -> Mux1/2, Transformation_BODY2GLOBAL/1
  Discrete-Time Integrator/1 -> Mux5/1  "PosVEH wrt  GLOB"

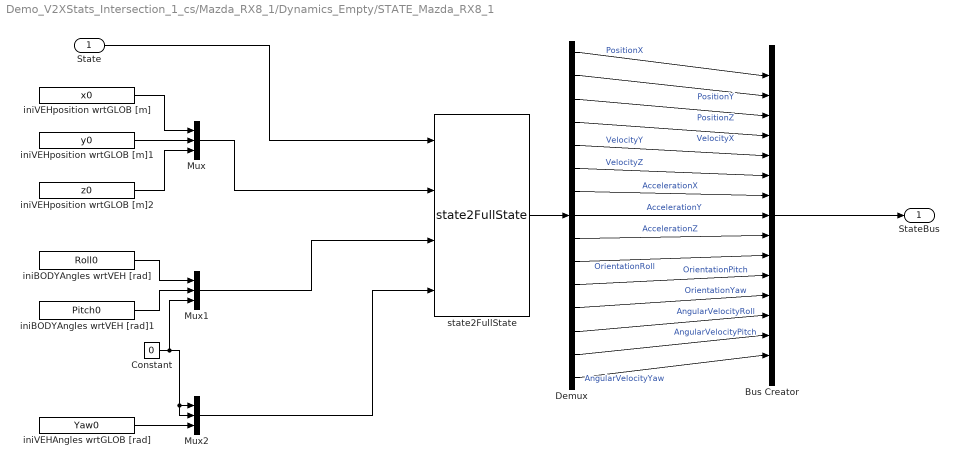
== system Demo_V2XStats_Intersection_1_cs/Mazda_RX8_1/Dynamics_Empty/STATE_Mazda_RX8_1 ==
  State : Inport  SampleTime=TimeStep
  Bus Creator : BusCreator  Inputs=15  OutDataTypeStr=Bus: PRESCAN_STATEACTUATORDATA  NonVirtualBus=on
  Constant : Constant  Value=0
  Demux : Demux  Outputs=15
  Mux : Mux  Inputs=3
  Mux1 : Mux  Inputs=3
  Mux2 : Mux  Inputs=3
  iniBODYAngles wrtVEH [rad] : Constant  Value=Roll0  SampleTime=TimeStep
  iniBODYAngles wrtVEH [rad]1 : Constant  Value=Pitch0  SampleTime=TimeStep
  iniVEHAngles wrtGLOB [rad] : Constant  Value=Yaw0  SampleTime=TimeStep
  iniVEHposition wrtGLOB [m] : Constant  Value=x0  SampleTime=TimeStep
  iniVEHposition wrtGLOB [m]1 : Constant  Value=y0  SampleTime=TimeStep
  iniVEHposition wrtGLOB [m]2 : Constant  Value=z0  SampleTime=TimeStep
  state2FullState : PreScanSimulinkLibrary/state2FullState  SystemSampleTime=-1
  StateBus : Outport  OutDataTypeStr=Bus: PRESCAN_STATEACTUATORDATA
  wires:
  Mux2/1 -> state2FullState/4
  iniVEHAngles wrtGLOB [rad]/1 -> Mux2/3
  Mux1/1 -> state2FullState/3
  Constant/1 -> Mux2/1, Mux2/2, Mux1/3
  iniBODYAngles wrtVEH [rad]1/1 -> Mux1/2
  iniBODYAngles wrtVEH [rad]/1 -> Mux1/1
  Mux/1 -> state2FullState/2
  iniVEHposition wrtGLOB [m]2/1 -> Mux/3
  iniVEHposition wrtGLOB [m]/1 -> Mux/1
  iniVEHposition wrtGLOB [m]1/1 -> Mux/2
  Demux/15 -> Bus Creator/15  "AngularVelocityYaw"
  Demux/14 -> Bus Creator/14  "AngularVelocityPitch"
  Demux/13 -> Bus Creator/13  "AngularVelocityRoll"
  Demux/12 -> Bus Creator/12  "OrientationYaw"
  Demux/11 -> Bus Creator/11  "OrientationPitch"
  Demux/10 -> Bus Creator/10  "OrientationRoll"
  Demux/9 -> Bus Creator/9  "AccelerationZ"
  Demux/8 -> Bus Creator/8  "AccelerationY"
  Demux/7 -> Bus Creator/7  "AccelerationX"
  Demux/6 -> Bus Creator/6  "VelocityZ"
  Demux/5 -> Bus Creator/5  "VelocityY"
  Demux/4 -> Bus Creator/4  "VelocityX"
  Demux/3 -> Bus Creator/3  "PositionZ"
  Demux/2 -> Bus Creator/2  "PositionY"
  Demux/1 -> Bus Creator/1  "PositionX"
  state2FullState/1 -> Demux/1
  State/1 -> state2FullState/1
  Bus Creator/1 -> StateBus/1

== system Demo_V2XStats_Intersection_1_cs/Mazda_RX8_1/SELF_Demux/compas converter ==
  rotz [rad] : Inport
  cart2compas : Subsystem
  rad2deg : Gain  Gain=180/pi
  heading [deg] : Outport
  wires:
  rad2deg/1 -> cart2compas/1(Angle [deg])
  rotz [rad]/1 -> rad2deg/1
  cart2compas/1(heading [deg]) -> heading [deg]/1

== system Demo_V2XStats_Intersection_1_cs/Mazda_RX8_1/Save_Plot_WarningData/warning hold ==
  warn : Inport
  Constant : Constant  Value=0
  Data Type Conversion1 : DataTypeConversion
  Data Type Conversion2 : DataTypeConversion
  Data Type Conversion3 : DataTypeConversion
  Discrete FIR Filter : DiscreteFir  Coefficients=0.1 * ones(1,10)  AccumDataTypeStr=Inherit: Same as product output
  Memory : Memory
  Switch : Switch  Criteria=u2 > Threshold
  Switch1 : Switch  Criteria=u2 ~= 0
  warning : Outport
  wires:
  Data Type Conversion3/1 -> warning/1
  Data Type Conversion2/1 -> Switch1/3
  Data Type Conversion1/1 -> Discrete FIR Filter/1, Switch/1, Switch/2
  Switch1/1 -> Data Type Conversion3/1
  Constant/1 -> Data Type Conversion2/1
  Discrete FIR Filter/1 -> Switch1/2
  Memory/1 -> Switch/3
  Switch/1 -> Switch1/1, Memory/1
  warn/1 -> Data Type Conversion1/1

== system Demo_V2XStats_Intersection_1_cs/Mazda_RX8_1/Save_Plot_WarningData/warning hold1 ==
  warn : Inport
  Constant : Constant  Value=0
  Data Type Conversion1 : DataTypeConversion
  Data Type Conversion2 : DataTypeConversion
  Data Type Conversion3 : DataTypeConversion
  Discrete FIR Filter : DiscreteFir  Coefficients=0.1 * ones(1,10)  AccumDataTypeStr=Inherit: Same as product output
  Memory : Memory
  Switch : Switch  Criteria=u2 > Threshold
  Switch1 : Switch  Criteria=u2 ~= 0
  warning : Outport
  wires:
  Data Type Conversion3/1 -> warning/1
  warn/1 -> Data Type Conversion1/1
  Switch/1 -> Memory/1, Switch1/1
  Memory/1 -> Switch/3
  Discrete FIR Filter/1 -> Switch1/2
  Constant/1 -> Data Type Conversion2/1
  Switch1/1 -> Data Type Conversion3/1
  Data Type Conversion1/1 -> Switch/2, Switch/1, Discrete FIR Filter/1
  Data Type Conversion2/1 -> Switch1/3

== system Demo_V2XStats_Intersection_1_cs/Mazda_RX8_1/Save_Plot_WarningData/warning hold2 ==
  warn : Inport
  Constant : Constant  Value=0
  Data Type Conversion1 : DataTypeConversion
  Data Type Conversion2 : DataTypeConversion
  Data Type Conversion3 : DataTypeConversion
  Discrete FIR Filter : DiscreteFir  Coefficients=0.1 * ones(1,10)  AccumDataTypeStr=Inherit: Same as product output
  Memory : Memory
  Switch : Switch  Criteria=u2 > Threshold
  Switch1 : Switch  Criteria=u2 ~= 0
  warning : Outport
  wires:
  Data Type Conversion3/1 -> warning/1
  Data Type Conversion2/1 -> Switch1/3
  Data Type Conversion1/1 -> Discrete FIR Filter/1, Switch/1, Switch/2
  Switch1/1 -> Data Type Conversion3/1
  Constant/1 -> Data Type Conversion2/1
  Discrete FIR Filter/1 -> Switch1/2
  Memory/1 -> Switch/3
  Switch/1 -> Switch1/1, Memory/1
  warn/1 -> Data Type Conversion1/1

== system Demo_V2XStats_Intersection_1_cs/Nissan_Cabstar_1/SELF_Demux/compas converter ==
  rotz [rad] : Inport
  cart2compas : Subsystem
  rad2deg : Gain  Gain=180/pi
  heading [deg] : Outport
  wires:
  rad2deg/1 -> cart2compas/1(Angle [deg])
  rotz [rad]/1 -> rad2deg/1
  cart2compas/1(heading [deg]) -> heading [deg]/1

== system Demo_V2XStats_Intersection_1_cs/Male_Regular_wSuitcase_1/SELF_Demux/compas converter/cart2compas ==
  Angle [deg] : Inport
  Constant : Constant  Value=90
  Constant1 : Constant  Value=360
  Gain : Gain  Gain=1/360
  Gain1 : Gain  Gain=360
  Gain2 : Gain  Gain=-1
  Rounding Function : Rounding
  Sum : Sum  Inputs=|-+
  Sum1 : Sum  Inputs=-+|
  Sum2 : Sum  Inputs=++|
  heading [deg] : Outport
  wires:
  Gain/1 -> Rounding Function/1
  Rounding Function/1 -> Gain1/1
  Gain1/1 -> Sum/1
  Angle [deg]/1 -> Sum1/2
  Sum/1 -> Gain2/1
  Sum1/1 -> Gain/1, Sum/2
  Constant/1 -> Sum1/1
  Gain2/1 -> Sum2/2
  Constant1/1 -> Sum2/1
  Sum2/1 -> heading [deg]/1

== system Demo_V2XStats_Intersection_1_cs/Mazda_RX8_1/SELF_Demux/compas converter/cart2compas ==
  Angle [deg] : Inport
  Constant : Constant  Value=90
  Constant1 : Constant  Value=360
  Gain : Gain  Gain=1/360
  Gain1 : Gain  Gain=360
  Gain2 : Gain  Gain=-1
  Rounding Function : Rounding
  Sum : Sum  Inputs=|-+
  Sum1 : Sum  Inputs=-+|
  Sum2 : Sum  Inputs=++|
  heading [deg] : Outport
  wires:
  Gain/1 -> Rounding Function/1
  Rounding Function/1 -> Gain1/1
  Gain1/1 -> Sum/1
  Angle [deg]/1 -> Sum1/2
  Sum/1 -> Gain2/1
  Sum1/1 -> Gain/1, Sum/2
  Constant/1 -> Sum1/1
  Gain2/1 -> Sum2/2
  Constant1/1 -> Sum2/1
  Sum2/1 -> heading [deg]/1

== system Demo_V2XStats_Intersection_1_cs/Nissan_Cabstar_1/SELF_Demux/compas converter/cart2compas ==
  Angle [deg] : Inport
  Constant : Constant  Value=90
  Constant1 : Constant  Value=360
  Gain : Gain  Gain=1/360
  Gain1 : Gain  Gain=360
  Gain2 : Gain  Gain=-1
  Rounding Function : Rounding
  Sum : Sum  Inputs=|-+
  Sum1 : Sum  Inputs=-+|
  Sum2 : Sum  Inputs=++|
  heading [deg] : Outport
  wires:
  Gain/1 -> Rounding Function/1
  Rounding Function/1 -> Gain1/1
  Gain1/1 -> Sum/1
  Angle [deg]/1 -> Sum1/2
  Sum/1 -> Gain2/1
  Sum1/1 -> Gain/1, Sum/2
  Constant/1 -> Sum1/1
  Gain2/1 -> Sum2/2
  Constant1/1 -> Sum2/1
  Sum2/1 -> heading [deg]/1

== stateflow chart Demo_V2XStats_Intersection_1_cs/Mazda_RX8_1/Decision Algorithm ==
  state Decision_algorithm
    state CAR1 [parallel]
      settings: executionOrder=1
      state Lane2
        state RightTurn
          en: W[2]=WM[4];
        state Straight
          en: W[2]=WM[5];
        state LeftTurn
          en: W[2]=WM[6];
        (default) -> (junction 123) [order 1]
        (junction 123) -> Decision_algorithm.CAR1.Lane2.LeftTurn [order 1] : [C1[3]<0]
        (junction 123) -> Decision_algorithm.CAR1.Lane2.RightTurn [order 3] : [C1[3]>0]
        (junction 123) -> Decision_algorithm.CAR1.Lane2.Straight [order 2] : [C1[3]==0]
        (default) -> Decision_algorithm.CAR1.Lane2.Straight [order 2]
      state Lane1
        state LeftTurn
          en: W[1]=WM[3];
        state Straight
          en: W[1]=WM[2];
        state RightTurn
          en: W[1]=WM[1];
        (junction 122) -> Decision_algorithm.CAR1.Lane1.LeftTurn [order 1] : [C1[3]<0]
        (default) -> (junction 122) [order 1]
        (junction 122) -> Decision_algorithm.CAR1.Lane1.Straight [order 2] : [C1[3]==0]
        (default) -> Decision_algorithm.CAR1.Lane1.Straight [order 2]
        (junction 122) -> Decision_algorithm.CAR1.Lane1.RightTurn [order 3] : [C1[3]>0]
      state Lane3
        state RightTurn
          en: W[3]=WM[7];
        state Straight
          en: W[3]=WM[8];
        state LeftTurn
          en: W[3]=WM[9];
        (junction 124) -> Decision_algorithm.CAR1.Lane3.RightTurn [order 1] : [C1[3]>0]
        (default) -> (junction 124) [order 1]
        (junction 124) -> Decision_algorithm.CAR1.Lane3.Straight [order 3] : [C1[3]==0]
        (junction 124) -> Decision_algorithm.CAR1.Lane3.LeftTurn [order 2] : [C1[3]<0]
        (default) -> Decision_algorithm.CAR1.Lane3.Straight [order 2]
      state Enter
      Decision_algorithm.CAR1.Lane2.RightTurn -> Enter
      Decision_algorithm.CAR1.Lane2.Straight -> Enter
      Decision_algorithm.CAR1.Lane2.LeftTurn -> Enter
      Enter -> Lane2 [order 1] : [C1[2]>-45 && C1[2]<0 && C1[1]<Rcross...
          | && C1[4]>225 && C1[4]<315]
      Enter -> Lane1 [order 3] : [C1[2]>45 && C1[2]<90 && C1[1]<Rcross...
          | && C1[4]>135 && C1[4]<225]
      Decision_algorithm.CAR1.Lane3.RightTurn -> Enter
      Decision_algorithm.CAR1.Lane1.LeftTurn -> Enter
      Decision_algorithm.CAR1.Lane3.Straight -> Enter
      Decision_algorithm.CAR1.Lane3.LeftTurn -> Enter
      Decision_algorithm.CAR1.Lane1.Straight -> Enter
      Enter -> Lane3 [order 2] : [C1[2]>-135 && C1[2]<-90 && C1[1]<Rcross...
          | && ((C1[4]>315 && C1[4]<=360) ||...
          | (C1[4]>=0 && C1[4]<45))]
      Decision_algorithm.CAR1.Lane1.RightTurn -> Enter
      Enter -> Enter [order 4] : {W[1]=0;
          | W[2]=0;
          | W[3]=0;}
      (default) -> Enter : {W[1]=0;
          | W[2]=0;
          | W[3]=0;}
  data: WM input size=9; Rcross input; C1 input size=4; W output boolean size=9

== matlab function Demo_V2XStats_Intersection_1_cs/Mazda_RX8_1/Select valid message ==
  data: u input Bus: PRESCAN_V2X_FIXED_CAM_MESSAGE; y output Bus: PRESCAN_V2X_FIXED_CAM_MESSAGE
function y = fcn(u)
%#codegen

y = u(1);

for k = 1 : numel(u)
    if u(k).HEADER.valid
        y = u(k);
        break
    end
end

== matlab function Demo_V2XStats_Intersection_1_cs/Mazda_RX8_1/Intention Conversion ==
  data: Intention_In input; Intention_Out output
function Intention_Out = fcn(Intention_In)
%#eml

Intention_Out = 0;

if Intention_In == 4
    Intention_Out = -1;
elseif Intention_In == 8
    Intention_Out = 1;
end

== matlab function Demo_V2XStats_Intersection_1_cs/Nissan_Cabstar_1/Date//Time Format Conversion ==
  data: Generation_Time_Epoch output
function Generation_Time_Epoch = Epoch_Time()

eml.extrinsic('now','datenum');

%Pre-allocate variables
Generation_Time = 0;
Reference_Time = 0;
Generation_Time_E = 0;

%Date/Time conversion
Generation_Time=datenum(now);                                     %Timezone - GMT+2
Reference_Time=datenum('20040101 020000.000','yyyymmdd HHMMSS');  %Reference Date/Time for the CAM/DENM - GMT/UTC
Generation_Time_E=round((Generation_Time-Reference_Time)*86400);  %Round to fix truncation

%Leap Seconds since 2004
Generation_Time_E = Generation_Time_E + 4;

Generation_Time_Epoch = int32(Generation_Time_E);
